simulink library "commanabbnd"  (Simulink 5.0)
values from neighbouring files (symbols this model uses):
  i = 0:length(h)-1    [commblkfadingchan.m]    (also in eyesampl.m = 3)
undefined symbols (not defined in the file or in its folder): den, num
libraries: commanabbnd x4, commutil x3
settings Model: Creator=tdelve  LastModifiedBy=mmclerno

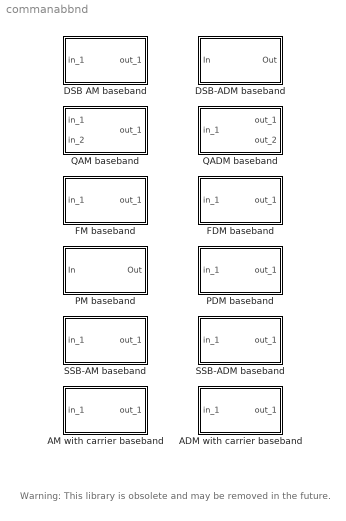
== system commanabbnd ==
  note: Warning:  This library is obsolete and may
      | be removed in the future.
  ADM with carrier baseband : Subsystem  mask(ADM with TC CE){Offset=1, num=[4.57 9.14 4.57]*.01, den=[1 -1.3108 .4936], Ph=0, ts=0.001}
      mask prompts: Offset "Output signal offset:"; num "Lowpass filter numerator:"; den "Lowpass filter denominator:"; Ph "Initial Phase (rad):"; ts "Sample time (ts):"
      mask help: Demodulate the complex envelope of an AM with TC modulated signal.
      mask Help: This block demodulates the complex envelope of an AM with transport carrier modulated signal. This block requires you to specify a lowpass filter, which eliminates the carrier frequency and keeps the message signal. This block takes a complex signal.
      mask Display:
      | plot(0,0,100,100,[5+4.5*[0:.3:10] 50 50 50 50+4.5*[0:10]],[85+10*[sin([0:.3:10]*pi/5).*sin([0:.3:10]*pi*2)] 85 99 75 10*sin([0:10]*pi/5)+85]);
      | disp('ADM w TC')
  AM with carrier baseband : Subsystem  mask(AM CE with TC){Offset=1, Ph=0}
      mask prompts: Offset "Input signal offset:"; Ph "Initial phase (rad):"
      mask help: Output complex envelope of an AM with transport carrier modulated signal.
      mask Help: This block causes the amplitude of the sinusoid carrier to depend on the message signal. An offset is added to the input signal before modulation. The output of this block is a complex signal. This modulation technique is not efficient.
      mask Display:
      | plot(0,0,100,100,[4.5*[0:10]+5 50 50 50 50+4.5*[0:.3:10]],[10*sin([0:10]*pi/5)+85 85 99 75 85+10*[sin([0:.3:10]*pi/5).*sin([0:.3:10]*pi*2)]]);
      | disp('AM w TC')
  DSB AM baseband : Subsystem  mask(DSB-SC AM CE){Ph=pi/2}
      mask prompts: Ph "Initial Phase (rad):"
      mask help: Output the complex envelope of a DSB-SC AM modulated signal.
      mask init:
      | x1=cos(Ph);x2=sin(Ph);pi2=2*pi;
      mask Help: This block outputs the complex envelope of the double-sideband suppressed-carrier amplitude modulated signal. The output is a complex signal.
      mask Display:
      | plot(0,0,100,100,[4.5*[0:10]+5 50 50 50 50+4.5*[0:.3:10]],[10*sin([0:10]*pi/5)+85 85 99 75 85+10*[sin([0:.3:10]*pi/5).*sin([0:.3:10]*pi*2)]]);
      | disp('DSB AM')
  DSB-ADM baseband : Subsystem  mask(DSB-SC ADM CE){num=[4.57 9.14 4.57]*.01, den=[1 -1.3108 .4936], Ph=pi/2, ts=0.001}
      mask prompts: num "Lowpass filter numerator:"; den "Lowpass filter denominator:"; Ph "Initial phase (rad):"; ts "Sample time (sec):"
      mask help: Demodulate the complex envelope of a DSB-SC AM modulated signal.
      mask init:
      | pi2=pi*2;
      mask Help: This block demodulates the complex envelope of a DSB-SC-AM modulated signal using Costas phase-locked loop method. This block requires you to specify a lowpass filter that eliminates the carrier frequency and keeps the message signal. This block takes a complex signal.
      mask Display:
      | plot(0,0,100,100,[5+4.5*[0:.3:10] 50 50 50 50+4.5*[0:10]],[85+10*[sin([0:.3:10]*pi/5).*sin([0:.3:10]*pi*2)] 85 99 75 10*sin([0:10]*pi/5)+85]);
      | disp('DSB ADM')
  FDM baseband : Subsystem  mask(FDM CE using PLL){Ph=0, HzPerVolt=1, num=[4.57 9.14 4.57]*.01, den=[1 -1.3108 .4936], ts=0.001}
      mask prompts: Ph "Initial phase (rad):"; HzPerVolt "Modulation constant (Hertz per volt):"; num "Lowpass filter numerator:"; den "Lowpass filter denominator:"; ts "Sample time (sec):"
      mask help: Demodulate the complex envelope of a FM signal.
      mask init:
      | pi2=2*pi;
      | Kc=2*pi*HzPerVolt;
      mask Help: This block demodulates the complex envelope of a frequency modulated signal. The filter to be specified by the users is a lowpass filter which passes the signal message and eliminates the carrier signal.
      mask Display:
      | plot(0,0,100,100,[5+4.5*[0:.15:10] 50 50 50 50+4.5*[0:10]],[85+10*[sin([0:.15:10]*pi*2+cumsum(sin([0:.15:10]*pi/5))/2)] 85 99 75   10*sin([0:10]*pi/5)+85]);
      | disp('FDM')
  FM baseband : Subsystem  mask(FM CE){Ph=0, HzPerV=1, ts=0.001, td=Inf}
      mask prompts: Ph "Initial phase (rad):"; HzPerV "Modulation constant (Hertz per volt):"; ts "Sample time (second):"; td "Symbol interval (for digital mod, use Inf for analog mod):"
      mask help: Output the complex envelope of the FM signal.
      mask init:
      | Kc =2*pi*HzPerV;if isinf(td),td=realmax;end;
      mask Help: This block outputs the complex envelope of the frequency modulated signal. The output is a complex signal. This block resets the phase at the very beginning of the symbol interval. For continuous-time simulation, the symbol interval can be set as infinity.
      mask Display:
      | plot(0,0,100,100,[4.5*[0:10]+5 50 50 50 50+4.5*[0:.15:10]],[10*sin([0:10]*pi/5)+85 85 99 75 85+10*[sin([0:.15:10]*pi*2+cumsum(sin([0:.15:10]*pi/5))/2)]]);
      | disp('FM')
  PDM baseband : Subsystem  mask(PLL PDM CE){Ph=0, Kc=1, num=[4.57 9.14 4.57]*.01, den=[1 -1.3108 .4936], HzPerVolt=1, ts=0.001}
      mask prompts: Ph "Initial phase (rad):"; Kc "Modulation constant (Radians per volt):"; num "Lowpass filter numerator:"; den "Lowpass filter denominator:"; HzPerVolt "VCO gain (Hertz per volt):"; ts "Sample time (sec):"
      mask help: Demodulate the complex envelope of a PM modulated signal.
      mask init:
      | Kv=2*pi*HzPerVolt;
      mask Help: This block demodulates the complex envelope of a PM modulated signal. This block uses a phase-locked loop with a multiplier phase detector.
      mask Display:
      | plot(0,0,100,100,[5+4.5*[0:.15:10] 50 50 50 50+4.5*[0:10]],[85+10*[sin([0:.15:10]*pi*2+cumsum(sin([0:.15:10]*pi/5))/2)] 85 99 75   10*sin([0:10]*pi/5)+85]);
      | disp('PDM')
  PM baseband : Subsystem  mask(PM CE){Ph=0, Kc=1}
      mask prompts: Ph "Initial phase (rad):"; Kc "Modulation constant (Radians per volt):"
      mask help: Output the complex envelope of a PM modulated signal.
      mask Help: This block outputs the complex envelope of the phase modulated signal. The output of this block is a complex signal.
      mask Display:
      | plot(0,0,100,100,[4.5*[0:10]+5 50 50 50 50+4.5*[0:.15:10]],[10*sin([0:10]*pi/5)+85 85 99 75 85+10*[sin([0:.15:10]*pi*2+cumsum(sin([0:.15:10]*pi/5))/2)]]);
      | disp('PM')
  QADM baseband : Subsystem  mask(QM DSB-SC ADM CE){num=[4.57 9.14 4.57]*.01, den=[1 -1.3108 .4936], Ph=0, ts=0.001}
      mask prompts: num "Lowpass filter numerator:"; den "Lowpass filter denominator:"; Ph "Initial phase (rad):"; ts "Sample time (sec):"
      mask help: Demodulate the complex envelope of a QAM modulated signal into in-phase and quadrature components into 1st and 2nd out ports.
      mask Help: This block demodulates the quadratic multiplexed double-sideband suppressed-carrier amplitude modulation modulated signal using the QAM method. The filter to be specified is a lowpass filter that passes the signal message and eliminates the carrier signal.
      mask Display:
      | plot(0,0,100,100,[5+4.5*[0:.3:10] 50 50 50 50+4.5*[0:10]],[85+10*[sin([0:.3:10]*pi/5).*sin([0:.3:10]*pi*2)] 85 99 75 10*sin([0:10]*pi/5)+85]);
      | disp('QADM')
  QAM baseband : Subsystem  mask(QM DSB-SC AM CE){Ph=0}
      mask prompts: Ph "Initial phase (rad):"
      mask help: Modulate the in-phase and quadrature component signal from the 1st and 2nd input ports, baseband simulation.
      mask Help: This block outputs the complex envelope of the quadratic multiplexed double-sideband suppressed-carrier amplitude modulated signal. The 1st and 2nd input ports input the in-phase and quadrature components. The output is a complex signal.
      mask Display:
      | plot(0,0,100,100,[4.5*[0:10]+5 50 50 50 50+4.5*[0:.3:10]],[10*sin([0:10]*pi/5)+85 85 99 75 85+10*[sin([0:.3:10]*pi/5).*sin([0:.3:10]*pi*2)]]);
      | disp('QAM')
  SSB-ADM baseband : Subsystem  mask(SSB-SC ADM CE){num=[4.57 9.14 4.57]*.01, den=[1 -1.3108 .4936], Ph=0, ts=0.001}
      mask prompts: num "Lowpass filter numerator:"; den "Lowpass filter denominator:"; Ph "Initial phase (rad):"; ts "Sample time (sec):"
      mask help: Demodulate the complex envelope of a SSB AM modulated signal.
      mask init:
      | x1=cos(-Ph);x2=sin(-Ph);
      mask Help: This block demodulates the complex envelope of a SSB-SC-AM modulated signal. This block requires you to specify a lowpass filter which eliminates the carrier frequency and keeps the message signal. This block takes a complex signal.
      mask Display:
      | plot(0,0,100,100,[5+4.5*[0:.3:10] 50 50 50 50+4.5*[0:10]],[85+10*[sin([0:.3:10]*pi/5).*sin([0:.3:10]*pi*2)] 85 99 75 10*sin([0:10]*pi/5)+85]);
      | disp('SSB ADM')
  SSB-AM baseband : Subsystem  mask(SSB-AM CE using Hilbert transform filter.){Ph=0, ban=10, dly=0.01, ts=0.001, sd='upper'}
      mask prompts: Ph "Initial Phase (rad):"; ban "Bandwidth of the input signal (Hz):"; dly "Time delay for Hilbert transform filter (sec):"; ts "Sample time (sec):"; sd ""upper" sideband or "lower" sideband:"
      mask help: Output complex envelope of a SSB AM modulated signal.
      mask init:
      | k=-1;if sd(1)=='l',k=1;end;if ban>1/ts, ban=1/ts-ts;end;[num,den]=hilbiir(ts,dly,ban);pi2=2*pi;pih=pi/2;
      mask Help: This block outputs the complex envelope of a SSB AM modulated signal. This block uses the Hilbert transfer filter. Because the Hilbert transform filter is a non-causal filter, you must use a positive time delay in the implementation. The input signal bandwidth is needed in designing the Hilbert transform filter. You can specify the modulation to be an USB or LSB modulation.
      mask Display:
      | plot(0,0,100,100,[4.5*[0:10]+5 50 50 50 50+4.5*[0:.3:10]],[10*sin([0:10]*pi/5)+85 85 99 75 85+10*[sin([0:.3:10]*pi/5).*sin([0:.3:10]*pi*2)]]);
      | disp('SSB AM')

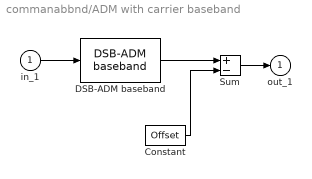
== system commanabbnd/ADM with carrier baseband ==
  in_1 : Inport
  Constant : Constant  Value=Offset
  DSB-ADM baseband : commanabbnd/DSB-ADM baseband  num=num  den=den  Ph=Ph  ts=ts
  Sum : Sum  Inputs=+-  SaturateOnIntegerOverflow=on  InputSameDT=on
  out_1 : Outport  InitialOutput=0
  wires:
  Sum/1 -> out_1/1
  DSB-ADM baseband/1 -> Sum/1
  in_1/1 -> DSB-ADM baseband/1
  Constant/1 -> Sum/2

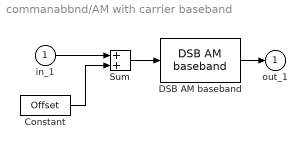
== system commanabbnd/AM with carrier baseband ==
  in_1 : Inport
  Constant : Constant  Value=Offset
  DSB AM baseband : commanabbnd/DSB AM baseband  Ph=Ph
  Sum : Sum  SaturateOnIntegerOverflow=on  InputSameDT=on
  out_1 : Outport  InitialOutput=0
  wires:
  Constant/1 -> Sum/2
  DSB AM baseband/1 -> out_1/1
  in_1/1 -> Sum/1
  Sum/1 -> DSB AM baseband/1

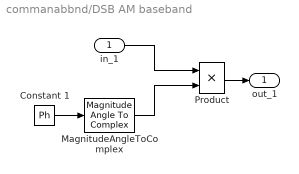
== system commanabbnd/DSB AM baseband ==
  in_1 : Inport
  Constant 1 : Constant  Value=Ph
  MagnitudeAngleToComplex : MagnitudeAngleToComplex  Input=Angle  ConstantPart=1
  Product : Product  SaturateOnIntegerOverflow=on  InputSameDT=on
  out_1 : Outport  InitialOutput=0
  wires:
  in_1/1 -> Product/1
  Product/1 -> out_1/1
  MagnitudeAngleToComplex/1 -> Product/2
  Constant 1/1 -> MagnitudeAngleToComplex/1

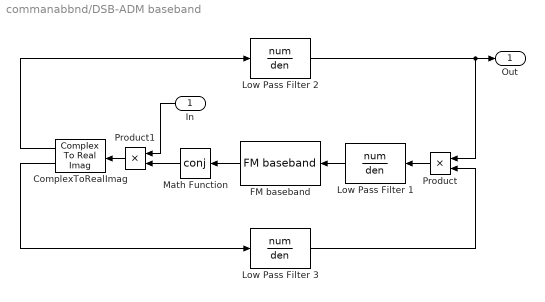
== system commanabbnd/DSB-ADM baseband ==
  In : Inport  Orientation=left
  ComplexToRealImag : ComplexToRealImag  Orientation=left
  FM baseband : commanabbnd/FM baseband  Orientation=left  Ph=Ph  HzPerV=1  ts=ts  td=Inf
  Low Pass Filter 1 : DiscreteFilter  Orientation=left  Numerator=num  Denominator=den  SampleTime=ts
  Low Pass Filter 2 : DiscreteFilter  Numerator=num  Denominator=den  SampleTime=ts
  Low Pass Filter 3 : DiscreteFilter  Numerator=num  Denominator=den  SampleTime=ts
  Math Function : Math  Orientation=left  Operator=conj
  Product : Product  Orientation=left  SaturateOnIntegerOverflow=on  InputSameDT=on
  Product1 : Product  Orientation=left  SaturateOnIntegerOverflow=on  InputSameDT=on
  Out : Outport  InitialOutput=0
  wires:
  ComplexToRealImag/1 -> Low Pass Filter 2/1
  ComplexToRealImag/2 -> Low Pass Filter 3/1
  Product/1 -> Low Pass Filter 1/1
  Product1/1 -> ComplexToRealImag/1
  In/1 -> Product1/1
  Math Function/1 -> Product1/2
  FM baseband/1 -> Math Function/1
  Low Pass Filter 3/1 -> Product/2
  Low Pass Filter 1/1 -> FM baseband/1
  Low Pass Filter 2/1 -> Product/1, Out/1

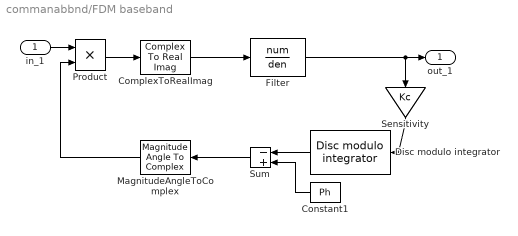
== system commanabbnd/FDM baseband ==
  in_1 : Inport
  ComplexToRealImag : ComplexToRealImag  Output=Imag
  Constant1 : Constant  Orientation=left  Value=Ph
  Disc modulo integrator : commutil/Disc modulo integrator  Orientation=left  modu=pi2  init=0  ts=ts
  Filter : DiscreteFilter  Numerator=num  Denominator=den  SampleTime=ts
  MagnitudeAngleToComplex : MagnitudeAngleToComplex  Orientation=left  Input=Angle  ConstantPart=1
  Product : Product  SaturateOnIntegerOverflow=on  InputSameDT=on
  Sensitivity : Gain  Orientation=down  Gain=Kc  SaturateOnIntegerOverflow=on
  Sum : Sum  Orientation=left  Inputs=-+  SaturateOnIntegerOverflow=on  InputSameDT=on
  out_1 : Outport  InitialOutput=0
  wires:
  Filter/1 -> Sensitivity/1, out_1/1
  in_1/1 -> Product/1
  Product/1 -> ComplexToRealImag/1
  ComplexToRealImag/1 -> Filter/1
  MagnitudeAngleToComplex/1 -> Product/2
  Sensitivity/1 -> Disc modulo integrator/1
  Disc modulo integrator/1 -> Sum/1
  Constant1/1 -> Sum/2
  Sum/1 -> MagnitudeAngleToComplex/1

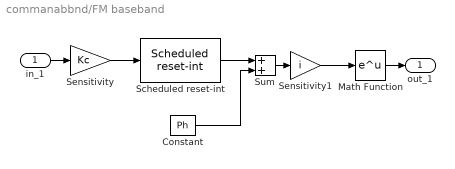
== system commanabbnd/FM baseband ==
  in_1 : Inport
  Constant : Constant  Value=Ph
  Math Function : Math
  Scheduled reset-int : commutil/Scheduled reset-int  td=td  ts=ts  limit=2*pi
  Sensitivity : Gain  Gain=Kc  SaturateOnIntegerOverflow=on
  Sensitivity1 : Gain  Gain=i  SaturateOnIntegerOverflow=on
  Sum : Sum  SaturateOnIntegerOverflow=on  InputSameDT=on
  out_1 : Outport  InitialOutput=0
  wires:
  Sensitivity/1 -> Scheduled reset-int/1
  in_1/1 -> Sensitivity/1
  Scheduled reset-int/1 -> Sum/1
  Constant/1 -> Sum/2
  Sum/1 -> Sensitivity1/1
  Sensitivity1/1 -> Math Function/1
  Math Function/1 -> out_1/1

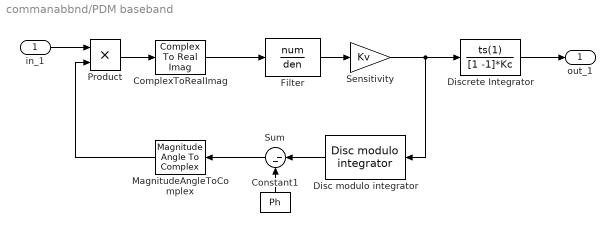
== system commanabbnd/PDM baseband ==
  in_1 : Inport
  ComplexToRealImag : ComplexToRealImag  Output=Imag
  Constant1 : Constant  Orientation=up  Value=Ph
  Disc modulo integrator : commutil/Disc modulo integrator  Orientation=left  modu=2*pi  init=0  ts=ts
  Discrete Integrator : DiscreteFilter  Numerator=ts(1)  Denominator=[1 -1]*Kc  SampleTime=ts
  Filter : DiscreteFilter  Numerator=num  Denominator=den  SampleTime=ts
  MagnitudeAngleToComplex : MagnitudeAngleToComplex  Orientation=left  Input=Angle  ConstantPart=1
  Product : Product  SaturateOnIntegerOverflow=on  InputSameDT=on
  Sensitivity : Gain  Gain=Kv  SaturateOnIntegerOverflow=on
  Sum : Sum  Orientation=left  Inputs=|--  SaturateOnIntegerOverflow=on  InputSameDT=on
  out_1 : Outport  InitialOutput=0
  wires:
  Discrete Integrator/1 -> out_1/1
  Sum/1 -> MagnitudeAngleToComplex/1
  Constant1/1 -> Sum/2
  Disc modulo integrator/1 -> Sum/1
  MagnitudeAngleToComplex/1 -> Product/2
  ComplexToRealImag/1 -> Filter/1
  Product/1 -> ComplexToRealImag/1
  in_1/1 -> Product/1
  Filter/1 -> Sensitivity/1
  Sensitivity/1 -> Discrete Integrator/1, Disc modulo integrator/1

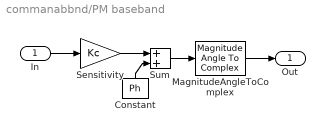
== system commanabbnd/PM baseband ==
  In : Inport
  Constant : Constant  Orientation=up  Value=Ph
  MagnitudeAngleToComplex : MagnitudeAngleToComplex  Input=Angle  ConstantPart=1
  Sensitivity : Gain  Gain=Kc  SaturateOnIntegerOverflow=on
  Sum : Sum  SaturateOnIntegerOverflow=on  InputSameDT=on
  Out : Outport  InitialOutput=0
  wires:
  In/1 -> Sensitivity/1
  Constant/1 -> Sum/2
  MagnitudeAngleToComplex/1 -> Out/1
  Sum/1 -> MagnitudeAngleToComplex/1
  Sensitivity/1 -> Sum/1

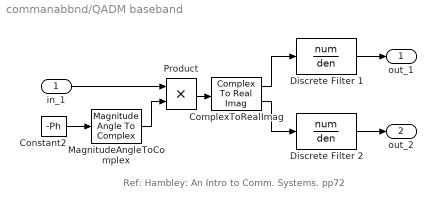
== system commanabbnd/QADM baseband ==
  note: Ref: Hambley: An Intro to Comm. Systems. pp72
  in_1 : Inport
  ComplexToRealImag : ComplexToRealImag
  Constant2 : Constant  Value=-Ph
  Discrete Filter 1 : DiscreteFilter  Numerator=num  Denominator=den  SampleTime=ts
  Discrete Filter 2 : DiscreteFilter  Numerator=num  Denominator=den  SampleTime=ts
  MagnitudeAngleToComplex : MagnitudeAngleToComplex  Input=Angle  ConstantPart=1
  Product : Product  SaturateOnIntegerOverflow=on  InputSameDT=on
  out_1 : Outport  InitialOutput=0
  out_2 : Outport  Port=2  InitialOutput=0
  wires:
  MagnitudeAngleToComplex/1 -> Product/2
  Constant2/1 -> MagnitudeAngleToComplex/1
  in_1/1 -> Product/1
  Product/1 -> ComplexToRealImag/1
  ComplexToRealImag/1 -> Discrete Filter 1/1
  Discrete Filter 1/1 -> out_1/1
  ComplexToRealImag/2 -> Discrete Filter 2/1
  Discrete Filter 2/1 -> out_2/1

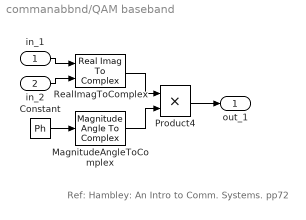
== system commanabbnd/QAM baseband ==
  note: Ref: Hambley: An Intro to Comm. Systems. pp72
  in_1 : Inport
  in_2 : Inport  Port=2
  Constant : Constant  Value=Ph
  MagnitudeAngleToComplex : MagnitudeAngleToComplex  Input=Angle  ConstantPart=1
  Product4 : Product  SaturateOnIntegerOverflow=on  InputSameDT=on
  RealImagToComplex : RealImagToComplex
  out_1 : Outport  InitialOutput=0
  wires:
  Product4/1 -> out_1/1
  in_1/1 -> RealImagToComplex/1
  in_2/1 -> RealImagToComplex/2
  RealImagToComplex/1 -> Product4/1
  Constant/1 -> MagnitudeAngleToComplex/1
  MagnitudeAngleToComplex/1 -> Product4/2

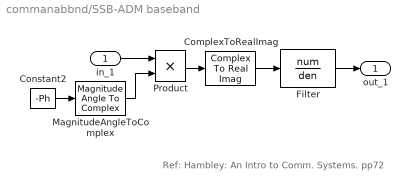
== system commanabbnd/SSB-ADM baseband ==
  note: Ref: Hambley: An Intro to Comm. Systems. pp72
  in_1 : Inport
  ComplexToRealImag : ComplexToRealImag  Output=Real
  Constant2 : Constant  Value=-Ph
  Filter : DiscreteFilter  Numerator=num  Denominator=den  SampleTime=ts
  MagnitudeAngleToComplex : MagnitudeAngleToComplex  Input=Angle  ConstantPart=1
  Product : Product  SaturateOnIntegerOverflow=on  InputSameDT=on
  out_1 : Outport  InitialOutput=0
  wires:
  Filter/1 -> out_1/1
  MagnitudeAngleToComplex/1 -> Product/2
  Constant2/1 -> MagnitudeAngleToComplex/1
  in_1/1 -> Product/1
  Product/1 -> ComplexToRealImag/1
  ComplexToRealImag/1 -> Filter/1

== system commanabbnd/SSB-AM baseband ==
  in_1 : Inport
  Filter : DiscreteFilter  Numerator=num  Denominator=den  SampleTime=ts
  Gain : Gain  Gain=k  SaturateOnIntegerOverflow=on
  QAM baseband : commanabbnd/QAM baseband  Ph=Ph
  out_1 : Outport  InitialOutput=0
  wires:
  Gain/1 -> QAM baseband/2
  Filter/1 -> Gain/1
  in_1/1 -> QAM baseband/1, Filter/1
  QAM baseband/1 -> out_1/1
